simulink library "xrbsComm_r3"  (Simulink 5.1)
libraries: xbsIndex_r3 x775, xrbsComm_r3 x1
(part 4 of 6)

== system xrbsComm_r3/White Gaussian  Noise Generator/Box-Muller3/fr1/lfsr_41_2/x5 ==
  " " : Inport
  reset : Inport  Port=2
  ASR : Subsystem  mask{init=[init(9) init(8) init(7) init(6) init(5) init(4) init(3) init(2) init(1)]}
      mask prompts: init "Initial Value"
      mask init:
      | init_size = size(init);
      | asr_length = init_size(2);
  Register : xbsIndex_r3/Register  init=init(10)  reg_only_valid=off  explicit_period=on  period=-1  rst=on  en=off  out_en=off  dbl_ovrd=off
      settings: xl_area=[0, 0, 0, 0, 0, 0, 0]
  z-10 : Outport
  wires:
  Register/1 -> ASR/1(din)
  ASR/1(dout) -> z-10/1
  " "/1 -> Register/1
  reset/1 -> Register/2

== system xrbsComm_r3/White Gaussian  Noise Generator/Box-Muller3/fr1/lfsr_41_2/x6 ==
  " " : Inport
  reset : Inport  Port=2
  ASR : Subsystem  mask{init=[init(8) init(7) init(6) init(5) init(4) init(3) init(2) init(1)]}
      mask prompts: init "Initial Value"
      mask init:
      | init_size = size(init);
      | asr_length = init_size(2);
  Register1 : xbsIndex_r3/Register  init=init(9)  reg_only_valid=off  explicit_period=on  period=-1  rst=on  en=off  out_en=off  dbl_ovrd=off
      settings: xl_area=[0, 0, 0, 0, 0, 0, 0]
  z-9 : Outport
  wires:
  ASR/1(dout) -> z-9/1
  " "/1 -> Register1/1
  Register1/1 -> ASR/1(din)
  reset/1 -> Register1/2

== system xrbsComm_r3/White Gaussian  Noise Generator/Box-Muller3/fr1/lfsr_41_2/x7 ==
  " " : Inport
  reset : Inport  Port=2
  ASR : Subsystem  mask{init=[init(8) init(7) init(6) init(5) init(4) init(3) init(2) init(1)]}
      mask prompts: init "Initial Value"
      mask init:
      | init_size = size(init);
      | asr_length = init_size(2);
  Register1 : xbsIndex_r3/Register  init=init(9)  reg_only_valid=off  explicit_period=on  period=-1  rst=on  en=off  out_en=off  dbl_ovrd=off
      settings: xl_area=[0, 0, 0, 0, 0, 0, 0]
  z-9 : Outport
  wires:
  ASR/1(dout) -> z-9/1
  Register1/1 -> ASR/1(din)
  " "/1 -> Register1/1
  reset/1 -> Register1/2

== system xrbsComm_r3/White Gaussian  Noise Generator/Box-Muller3/g2/lfsr_47_5/x10 ==
  "  " : Inport
  reset : Inport  Port=2
  ASR : Subsystem  mask{init=[init(4) init(3) init(2) init(1)]}
      mask prompts: init "Initial Value"
      mask init:
      | init_size = size(init);
      | asr_length = init_size(2);
  Register5 : xbsIndex_r3/Register  init=init(5)  reg_only_valid=off  explicit_period=on  period=-1  rst=on  en=off  out_en=off  dbl_ovrd=off
      settings: xl_area=[0, 0, 0, 0, 0, 0, 0]
  z-5 : Outport
  wires:
  ASR/1(dout) -> z-5/1
  Register5/1 -> ASR/1(din)
  "  "/1 -> Register5/1
  reset/1 -> Register5/2

== system xrbsComm_r3/White Gaussian  Noise Generator/Box-Muller3/g2/lfsr_47_5/x11 ==
  " " : Inport
  reset : Inport  Port=2
  ASR : Subsystem  mask{init=[init(4) init(3) init(2) init(1)]}
      mask prompts: init "Initial Value"
      mask init:
      | init_size = size(init);
      | asr_length = init_size(2);
  Register : xbsIndex_r3/Register  init=init(5)  reg_only_valid=off  explicit_period=on  period=-1  rst=on  en=off  out_en=off  dbl_ovrd=off
      settings: xl_area=[0, 0, 0, 0, 0, 0, 0]
  z-5 : Outport
  wires:
  ASR/1(dout) -> z-5/1
  Register/1 -> ASR/1(din)
  " "/1 -> Register/1
  reset/1 -> Register/2

== system xrbsComm_r3/White Gaussian  Noise Generator/Box-Muller3/g2/lfsr_47_5/x12 ==
  " " : Inport
  reset : Inport  Port=2
  ASR : Subsystem  mask{init=[init(4) init(3) init(2) init(1)]}
      mask prompts: init "Initial Value"
      mask init:
      | init_size = size(init);
      | asr_length = init_size(2);
  Register : xbsIndex_r3/Register  init=init(5)  reg_only_valid=off  explicit_period=on  period=-1  rst=on  en=off  out_en=off  dbl_ovrd=off
      settings: xl_area=[0, 0, 0, 0, 0, 0, 0]
  z-5 : Outport
  wires:
  ASR/1(dout) -> z-5/1
  Register/1 -> ASR/1(din)
  " "/1 -> Register/1
  reset/1 -> Register/2

== system xrbsComm_r3/White Gaussian  Noise Generator/Box-Muller3/g2/lfsr_47_5/x13 ==
  note: reset
  " " : Inport
  " 1" : Inport  Port=2
  ASR : Subsystem  mask{init=[init(4) init(3) init(2) init(1)]}
      mask prompts: init "Initial Value"
      mask init:
      | init_size = size(init);
      | asr_length = init_size(2);
  Register : xbsIndex_r3/Register  init=init(5)  reg_only_valid=off  explicit_period=on  period=-1  rst=on  en=off  out_en=off  dbl_ovrd=off
      settings: xl_area=[0, 0, 0, 0, 0, 0, 0]
  z-5 : Outport
  wires:
  ASR/1(dout) -> z-5/1
  Register/1 -> ASR/1(din)
  " "/1 -> Register/1
  " 1"/1 -> Register/2

== system xrbsComm_r3/White Gaussian  Noise Generator/Box-Muller3/g2/lfsr_47_5/x14 ==
  " " : Inport
  reset : Inport  Port=2
  ASR : Subsystem  mask{init=[init(4) init(3) init(2) init(1)]}
      mask prompts: init "Initial Value"
      mask init:
      | init_size = size(init);
      | asr_length = init_size(2);
  Register : xbsIndex_r3/Register  init=init(5)  reg_only_valid=off  explicit_period=on  period=-1  rst=on  en=off  out_en=off  dbl_ovrd=off
      settings: xl_area=[0, 0, 0, 0, 0, 0, 0]
  z-5 : Outport
  wires:
  ASR/1(dout) -> z-5/1
  Register/1 -> ASR/1(din)
  " "/1 -> Register/1
  reset/1 -> Register/2

== system xrbsComm_r3/White Gaussian  Noise Generator/Box-Muller3/g2/lfsr_47_5/x15 ==
  " " : Inport
  reset : Inport  Port=2
  ASR : Subsystem  mask{init=[init(4) init(3) init(2) init(1)]}
      mask prompts: init "Initial Value"
      mask init:
      | init_size = size(init);
      | asr_length = init_size(2);
  Register : xbsIndex_r3/Register  init=init(5)  reg_only_valid=off  explicit_period=on  period=-1  rst=on  en=off  out_en=off  dbl_ovrd=off
      settings: xl_area=[0, 0, 0, 0, 0, 0, 0]
  z-5 : Outport
  wires:
  ASR/1(dout) -> z-5/1
  Register/1 -> ASR/1(din)
  " "/1 -> Register/1
  reset/1 -> Register/2

== system xrbsComm_r3/White Gaussian  Noise Generator/Box-Muller3/g2/lfsr_47_5/x16 ==
  " " : Inport
  reset : Inport  Port=2
  ASR : Subsystem  mask{init=[init(3) init(2) init(1)]}
      mask prompts: init "Initial Value"
      mask init:
      | init_size = size(init);
      | asr_length = init_size(2);
  Register : xbsIndex_r3/Register  init=init(4)  reg_only_valid=off  explicit_period=on  period=-1  rst=on  en=off  out_en=off  dbl_ovrd=off
      settings: xl_area=[0, 0, 0, 0, 0, 0, 0]
  z-4 : Outport
  wires:
  ASR/1(dout) -> z-4/1
  Register/1 -> ASR/1(din)
  " "/1 -> Register/1
  reset/1 -> Register/2

== system xrbsComm_r3/White Gaussian  Noise Generator/Box-Muller3/g2/lfsr_47_5/x9 ==
  " " : Inport
  reset : Inport  Port=2
  ASR : Subsystem  mask{init=[init(4) init(3) init(2) init(1)]}
      mask prompts: init "Initial Value"
      mask init:
      | init_size = size(init);
      | asr_length = init_size(2);
  Register : xbsIndex_r3/Register  init=init(5)  reg_only_valid=off  explicit_period=on  period=-1  rst=on  en=off  out_en=off  dbl_ovrd=off
      settings: xl_area=[0, 0, 0, 0, 0, 0, 0]
  z-5 : Outport
  wires:
  ASR/1(dout) -> z-5/1
  Register/1 -> ASR/1(din)
  " "/1 -> Register/1
  reset/1 -> Register/2

== system xrbsComm_r3/White Gaussian  Noise Generator/Box-Muller4/fr1/lfsr_17_2/x1 ==
  " " : Inport
  " reset" : Inport  Port=2
  ASR : Subsystem  mask{init=[init(2) init(1)]}
      mask prompts: init "Initial Value"
      mask init:
      | init_size = size(init);
      | asr_length = init_size(2);
  Register4 : xbsIndex_r3/Register  init=init(3)  reg_only_valid=off  explicit_period=on  period=-1  rst=on  en=off  out_en=off  dbl_ovrd=off
      settings: xl_area=[0, 0, 0, 0, 0, 0, 0]
  z-3 : Outport
  wires:
  " "/1 -> Register4/1
  ASR/1(dout) -> z-3/1
  Register4/1 -> ASR/1(din)
  " reset"/1 -> Register4/2

== system xrbsComm_r3/White Gaussian  Noise Generator/Box-Muller4/fr1/lfsr_17_2/x5 ==
  " " : Inport
  reset : Inport  Port=2
  ASR : Subsystem  mask{init=[init(3) init(2) init(1)]}
      mask prompts: init "Initial Value"
      mask init:
      | init_size = size(init);
      | asr_length = init_size(2);
  Register5 : xbsIndex_r3/Register  init=init(4)  reg_only_valid=off  explicit_period=on  period=-1  rst=on  en=off  out_en=off  dbl_ovrd=off
      settings: xl_area=[0, 0, 0, 0, 0, 0, 0]
  z-4 : Outport
  wires:
  ASR/1(dout) -> z-4/1
  Register5/1 -> ASR/1(din)
  " "/1 -> Register5/1
  reset/1 -> Register5/2

== system xrbsComm_r3/White Gaussian  Noise Generator/Box-Muller4/fr1/lfsr_17_2/x6 ==
  " " : Inport
  " reset" : Inport  Port=2
  ASR : Subsystem  mask{init=[init(2) init(1)]}
      mask prompts: init "Initial Value"
      mask init:
      | init_size = size(init);
      | asr_length = init_size(2);
  Register4 : xbsIndex_r3/Register  init=init(3)  reg_only_valid=off  explicit_period=on  period=-1  rst=on  en=off  out_en=off  dbl_ovrd=off
      settings: xl_area=[0, 0, 0, 0, 0, 0, 0]
  z-3 : Outport
  wires:
  ASR/1(dout) -> z-3/1
  " "/1 -> Register4/1
  Register4/1 -> ASR/1(din)
  " reset"/1 -> Register4/2

== system xrbsComm_r3/White Gaussian  Noise Generator/Box-Muller4/fr1/lfsr_17_2/x7 ==
  " " : Inport
  reset : Inport  Port=2
  ASR : Subsystem  mask{init=[init(2) init(1)]}
      mask prompts: init "Initial Value"
      mask init:
      | init_size = size(init);
      | asr_length = init_size(2);
  Register4 : xbsIndex_r3/Register  init=init(3)  reg_only_valid=off  explicit_period=on  period=-1  rst=on  en=off  out_en=off  dbl_ovrd=off
      settings: xl_area=[0, 0, 0, 0, 0, 0, 0]
  z-3 : Outport
  wires:
  " "/1 -> Register4/1
  ASR/1(dout) -> z-3/1
  Register4/1 -> ASR/1(din)
  reset/1 -> Register4/2

== system xrbsComm_r3/White Gaussian  Noise Generator/Box-Muller4/fr1/lfsr_25_2/x1 ==
  " " : Inport
  reset : Inport  Port=2
  ASR : Subsystem  mask{init=[init(4) init(3) init(2) init(1)]}
      mask prompts: init "Initial Value"
      mask init:
      | init_size = size(init);
      | asr_length = init_size(2);
  Register : xbsIndex_r3/Register  init=init(5)  reg_only_valid=off  explicit_period=on  period=-1  rst=on  en=off  out_en=off  dbl_ovrd=off
      settings: xl_area=[0, 0, 0, 0, 0, 0, 0]
  z-5 : Outport
  wires:
  Register/1 -> ASR/1(din)
  ASR/1(dout) -> z-5/1
  " "/1 -> Register/1
  reset/1 -> Register/2

== system xrbsComm_r3/White Gaussian  Noise Generator/Box-Muller4/fr1/lfsr_25_2/x5 ==
  " " : Inport
  reset : Inport  Port=2
  ASR : Subsystem  mask{init=[init(5) init(4) init(3) init(2) init(1)]}
      mask prompts: init "Initial Value"
      mask init:
      | init_size = size(init);
      | asr_length = init_size(2);
  Register : xbsIndex_r3/Register  init=init(6)  reg_only_valid=off  explicit_period=on  period=-1  rst=on  en=off  out_en=off  dbl_ovrd=off
      settings: xl_area=[0, 0, 0, 0, 0, 0, 0]
  z-6 : Outport
  wires:
  Register/1 -> ASR/1(din)
  ASR/1(dout) -> z-6/1
  " "/1 -> Register/1
  reset/1 -> Register/2

== system xrbsComm_r3/White Gaussian  Noise Generator/Box-Muller4/fr1/lfsr_25_2/x6 ==
  " " : Inport
  reset : Inport  Port=2
  ASR : Subsystem  mask{init=[init(4) init(3) init(2) init(1)]}
      mask prompts: init "Initial Value"
      mask init:
      | init_size = size(init);
      | asr_length = init_size(2);
  Register : xbsIndex_r3/Register  init=init(5)  reg_only_valid=off  explicit_period=on  period=-1  rst=on  en=off  out_en=off  dbl_ovrd=off
      settings: xl_area=[0, 0, 0, 0, 0, 0, 0]
  z-5 : Outport
  wires:
  Register/1 -> ASR/1(din)
  ASR/1(dout) -> z-5/1
  " "/1 -> Register/1
  reset/1 -> Register/2

== system xrbsComm_r3/White Gaussian  Noise Generator/Box-Muller4/fr1/lfsr_25_2/x7 ==
  " " : Inport
  reset : Inport  Port=2
  ASR : Subsystem  mask{init=[init(4) init(3) init(2) init(1)]}
      mask prompts: init "Initial Value"
      mask init:
      | init_size = size(init);
      | asr_length = init_size(2);
  Register : xbsIndex_r3/Register  init=init(5)  reg_only_valid=off  explicit_period=on  period=-1  rst=on  en=off  out_en=off  dbl_ovrd=off
      settings: xl_area=[0, 0, 0, 0, 0, 0, 0]
  z-5 : Outport
  wires:
  Register/1 -> ASR/1(din)
  ASR/1(dout) -> z-5/1
  " "/1 -> Register/1
  reset/1 -> Register/2

== system xrbsComm_r3/White Gaussian  Noise Generator/Box-Muller4/fr1/lfsr_29_2/x5 ==
  " " : Inport
  reset : Inport  Port=2
  ASR : Subsystem  mask{init=[init(6) init(5) init(4) init(3) init(2) init(1)]}
      mask prompts: init "Initial Value"
      mask init:
      | init_size = size(init);
      | asr_length = init_size(2);
  Register : xbsIndex_r3/Register  init=init(7)  reg_only_valid=off  explicit_period=on  period=-1  rst=on  en=off  out_en=off  dbl_ovrd=off
      settings: xl_area=[0, 0, 0, 0, 0, 0, 0]
  z-7 : Outport
  wires:
  ASR/1(dout) -> z-7/1
  Register/1 -> ASR/1(din)
  " "/1 -> Register/1
  reset/1 -> Register/2

== system xrbsComm_r3/White Gaussian  Noise Generator/Box-Muller4/fr1/lfsr_29_2/x6 ==
  " " : Inport
  reset : Inport  Port=2
  ASR : Subsystem  mask{init=[init(5) init(4) init(3) init(2) init(1)]}
      mask prompts: init "Initial Value"
      mask init:
      | init_size = size(init);
      | asr_length = init_size(2);
  Register : xbsIndex_r3/Register  init=init(6)  reg_only_valid=off  explicit_period=on  period=-1  rst=on  en=off  out_en=off  dbl_ovrd=off
      settings: xl_area=[0, 0, 0, 0, 0, 0, 0]
  z-6 : Outport
  wires:
  ASR/1(dout) -> z-6/1
  Register/1 -> ASR/1(din)
  " "/1 -> Register/1
  reset/1 -> Register/2

== system xrbsComm_r3/White Gaussian  Noise Generator/Box-Muller4/fr1/lfsr_29_2/x7 ==
  " " : Inport
  reset : Inport  Port=2
  ASR : Subsystem  mask{init=[init(5) init(4) init(3) init(2) init(1)]}
      mask prompts: init "Initial Value"
      mask init:
      | init_size = size(init);
      | asr_length = init_size(2);
  Register : xbsIndex_r3/Register  init=init(6)  reg_only_valid=off  explicit_period=on  period=-1  rst=on  en=off  out_en=off  dbl_ovrd=off
      settings: xl_area=[0, 0, 0, 0, 0, 0, 0]
  z-6 : Outport
  wires:
  ASR/1(dout) -> z-6/1
  Register/1 -> ASR/1(din)
  " "/1 -> Register/1
  reset/1 -> Register/2

== system xrbsComm_r3/White Gaussian  Noise Generator/Box-Muller4/fr1/lfsr_29_2/x8 ==
  " " : Inport
  reset : Inport  Port=2
  ASR : Subsystem  mask{init=[init(5) init(4) init(3) init(2) init(1)]}
      mask prompts: init "Initial Value"
      mask init:
      | init_size = size(init);
      | asr_length = init_size(2);
  Register : xbsIndex_r3/Register  init=init(6)  reg_only_valid=off  explicit_period=on  period=-1  rst=on  en=off  out_en=off  dbl_ovrd=off
      settings: xl_area=[0, 0, 0, 0, 0, 0, 0]
  z-6 : Outport
  wires:
  ASR/1(dout) -> z-6/1
  Register/1 -> ASR/1(din)
  " "/1 -> Register/1
  reset/1 -> Register/2

== system xrbsComm_r3/White Gaussian  Noise Generator/Box-Muller4/fr1/lfsr_31_2/x5 ==
  " " : Inport
  reset : Inport  Port=2
  ASR : Subsystem  mask{init=[init(6) init(5) init(4) init(3) init(2) init(1)]}
      mask prompts: init "Initial Value"
      mask init:
      | init_size = size(init);
      | asr_length = init_size(2);
  Register : xbsIndex_r3/Register  init=init(7)  reg_only_valid=off  explicit_period=on  period=-1  rst=on  en=off  out_en=off  dbl_ovrd=off
      settings: xl_area=[0, 0, 0, 0, 0, 0, 0]
  z-7 : Outport
  wires:
  Register/1 -> ASR/1(din)
  ASR/1(dout) -> z-7/1
  " "/1 -> Register/1
  reset/1 -> Register/2

== system xrbsComm_r3/White Gaussian  Noise Generator/Box-Muller4/fr1/lfsr_31_2/x6 ==
  " " : Inport
  reset : Inport  Port=2
  ASR : Subsystem  mask{init=[init(6) init(5) init(4) init(3) init(2) init(1)]}
      mask prompts: init "Initial Value"
      mask init:
      | init_size = size(init);
      | asr_length = init_size(2);
  Register : xbsIndex_r3/Register  init=init(7)  reg_only_valid=off  explicit_period=on  period=-1  rst=on  en=off  out_en=off  dbl_ovrd=off
      settings: xl_area=[0, 0, 0, 0, 0, 0, 0]
  z-7 : Outport
  wires:
  Register/1 -> ASR/1(din)
  " "/1 -> Register/1
  ASR/1(dout) -> z-7/1
  reset/1 -> Register/2

== system xrbsComm_r3/White Gaussian  Noise Generator/Box-Muller4/fr1/lfsr_31_2/x7 ==
  " " : Inport
  reset : Inport  Port=2
  ASR : Subsystem  mask{init=[init(6) init(5) init(4) init(3) init(2) init(1)]}
      mask prompts: init "Initial Value"
      mask init:
      | init_size = size(init);
      | asr_length = init_size(2);
  Register : xbsIndex_r3/Register  init=init(7)  reg_only_valid=off  explicit_period=on  period=-1  rst=on  en=off  out_en=off  dbl_ovrd=off
      settings: xl_area=[0, 0, 0, 0, 0, 0, 0]
  z-7 : Outport
  wires:
  Register/1 -> ASR/1(din)
  ASR/1(dout) -> z-7/1
  " "/1 -> Register/1
  reset/1 -> Register/2

== system xrbsComm_r3/White Gaussian  Noise Generator/Box-Muller4/fr1/lfsr_31_2/x8 ==
  " " : Inport
  reset : Inport  Port=2
  ASR : Subsystem  mask{init=[init(5) init(4) init(3) init(2) init(1)]}
      mask prompts: init "Initial Value"
      mask init:
      | init_size = size(init);
      | asr_length = init_size(2);
  Register : xbsIndex_r3/Register  init=init(6)  reg_only_valid=off  explicit_period=on  period=-1  rst=on  en=off  out_en=off  dbl_ovrd=off
      settings: xl_area=[0, 0, 0, 0, 0, 0, 0]
  z-6 : Outport
  wires:
  Register/1 -> ASR/1(din)
  " "/1 -> Register/1
  ASR/1(dout) -> z-6/1
  reset/1 -> Register/2

== system xrbsComm_r3/White Gaussian  Noise Generator/Box-Muller4/fr1/lfsr_41_2/x1 ==
  " " : Inport
  reset : Inport  Port=2
  ASR : Subsystem  mask{init=[init(8) init(7) init(6) init(5) init(4) init(3) init(2) init(1)]}
      mask prompts: init "Initial Value"
      mask init:
      | init_size = size(init);
      | asr_length = init_size(2);
  Register1 : xbsIndex_r3/Register  init=init(9)  reg_only_valid=off  explicit_period=on  period=-1  rst=on  en=off  out_en=off  dbl_ovrd=off
      settings: xl_area=[0, 0, 0, 0, 0, 0, 0]
  z-9 : Outport
  wires:
  ASR/1(dout) -> z-9/1
  " "/1 -> Register1/1
  Register1/1 -> ASR/1(din)
  reset/1 -> Register1/2

== system xrbsComm_r3/White Gaussian  Noise Generator/Box-Muller4/fr1/lfsr_41_2/x5 ==
  " " : Inport
  reset : Inport  Port=2
  ASR : Subsystem  mask{init=[init(9) init(8) init(7) init(6) init(5) init(4) init(3) init(2) init(1)]}
      mask prompts: init "Initial Value"
      mask init:
      | init_size = size(init);
      | asr_length = init_size(2);
  Register : xbsIndex_r3/Register  init=init(10)  reg_only_valid=off  explicit_period=on  period=-1  rst=on  en=off  out_en=off  dbl_ovrd=off
      settings: xl_area=[0, 0, 0, 0, 0, 0, 0]
  z-10 : Outport
  wires:
  Register/1 -> ASR/1(din)
  ASR/1(dout) -> z-10/1
  " "/1 -> Register/1
  reset/1 -> Register/2

== system xrbsComm_r3/White Gaussian  Noise Generator/Box-Muller4/fr1/lfsr_41_2/x6 ==
  " " : Inport
  reset : Inport  Port=2
  ASR : Subsystem  mask{init=[init(8) init(7) init(6) init(5) init(4) init(3) init(2) init(1)]}
      mask prompts: init "Initial Value"
      mask init:
      | init_size = size(init);
      | asr_length = init_size(2);
  Register1 : xbsIndex_r3/Register  init=init(9)  reg_only_valid=off  explicit_period=on  period=-1  rst=on  en=off  out_en=off  dbl_ovrd=off
      settings: xl_area=[0, 0, 0, 0, 0, 0, 0]
  z-9 : Outport
  wires:
  ASR/1(dout) -> z-9/1
  " "/1 -> Register1/1
  Register1/1 -> ASR/1(din)
  reset/1 -> Register1/2

== system xrbsComm_r3/White Gaussian  Noise Generator/Box-Muller4/fr1/lfsr_41_2/x7 ==
  " " : Inport
  reset : Inport  Port=2
  ASR : Subsystem  mask{init=[init(8) init(7) init(6) init(5) init(4) init(3) init(2) init(1)]}
      mask prompts: init "Initial Value"
      mask init:
      | init_size = size(init);
      | asr_length = init_size(2);
  Register1 : xbsIndex_r3/Register  init=init(9)  reg_only_valid=off  explicit_period=on  period=-1  rst=on  en=off  out_en=off  dbl_ovrd=off
      settings: xl_area=[0, 0, 0, 0, 0, 0, 0]
  z-9 : Outport
  wires:
  ASR/1(dout) -> z-9/1
  Register1/1 -> ASR/1(din)
  " "/1 -> Register1/1
  reset/1 -> Register1/2

== system xrbsComm_r3/White Gaussian  Noise Generator/Box-Muller4/g2/lfsr_47_5/x10 ==
  "  " : Inport
  reset : Inport  Port=2
  ASR : Subsystem  mask{init=[init(4) init(3) init(2) init(1)]}
      mask prompts: init "Initial Value"
      mask init:
      | init_size = size(init);
      | asr_length = init_size(2);
  Register5 : xbsIndex_r3/Register  init=init(5)  reg_only_valid=off  explicit_period=on  period=-1  rst=on  en=off  out_en=off  dbl_ovrd=off
      settings: xl_area=[0, 0, 0, 0, 0, 0, 0]
  z-5 : Outport
  wires:
  ASR/1(dout) -> z-5/1
  Register5/1 -> ASR/1(din)
  "  "/1 -> Register5/1
  reset/1 -> Register5/2

== system xrbsComm_r3/White Gaussian  Noise Generator/Box-Muller4/g2/lfsr_47_5/x11 ==
  " " : Inport
  reset : Inport  Port=2
  ASR : Subsystem  mask{init=[init(4) init(3) init(2) init(1)]}
      mask prompts: init "Initial Value"
      mask init:
      | init_size = size(init);
      | asr_length = init_size(2);
  Register : xbsIndex_r3/Register  init=init(5)  reg_only_valid=off  explicit_period=on  period=-1  rst=on  en=off  out_en=off  dbl_ovrd=off
      settings: xl_area=[0, 0, 0, 0, 0, 0, 0]
  z-5 : Outport
  wires:
  ASR/1(dout) -> z-5/1
  Register/1 -> ASR/1(din)
  " "/1 -> Register/1
  reset/1 -> Register/2

== system xrbsComm_r3/White Gaussian  Noise Generator/Box-Muller4/g2/lfsr_47_5/x12 ==
  " " : Inport
  reset : Inport  Port=2
  ASR : Subsystem  mask{init=[init(4) init(3) init(2) init(1)]}
      mask prompts: init "Initial Value"
      mask init:
      | init_size = size(init);
      | asr_length = init_size(2);
  Register : xbsIndex_r3/Register  init=init(5)  reg_only_valid=off  explicit_period=on  period=-1  rst=on  en=off  out_en=off  dbl_ovrd=off
      settings: xl_area=[0, 0, 0, 0, 0, 0, 0]
  z-5 : Outport
  wires:
  ASR/1(dout) -> z-5/1
  Register/1 -> ASR/1(din)
  " "/1 -> Register/1
  reset/1 -> Register/2

== system xrbsComm_r3/White Gaussian  Noise Generator/Box-Muller4/g2/lfsr_47_5/x13 ==
  note: reset
  " " : Inport
  " 1" : Inport  Port=2
  ASR : Subsystem  mask{init=[init(4) init(3) init(2) init(1)]}
      mask prompts: init "Initial Value"
      mask init:
      | init_size = size(init);
      | asr_length = init_size(2);
  Register : xbsIndex_r3/Register  init=init(5)  reg_only_valid=off  explicit_period=on  period=-1  rst=on  en=off  out_en=off  dbl_ovrd=off
      settings: xl_area=[0, 0, 0, 0, 0, 0, 0]
  z-5 : Outport
  wires:
  ASR/1(dout) -> z-5/1
  Register/1 -> ASR/1(din)
  " "/1 -> Register/1
  " 1"/1 -> Register/2

== system xrbsComm_r3/White Gaussian  Noise Generator/Box-Muller4/g2/lfsr_47_5/x14 ==
  " " : Inport
  reset : Inport  Port=2
  ASR : Subsystem  mask{init=[init(4) init(3) init(2) init(1)]}
      mask prompts: init "Initial Value"
      mask init:
      | init_size = size(init);
      | asr_length = init_size(2);
  Register : xbsIndex_r3/Register  init=init(5)  reg_only_valid=off  explicit_period=on  period=-1  rst=on  en=off  out_en=off  dbl_ovrd=off
      settings: xl_area=[0, 0, 0, 0, 0, 0, 0]
  z-5 : Outport
  wires:
  ASR/1(dout) -> z-5/1
  Register/1 -> ASR/1(din)
  " "/1 -> Register/1
  reset/1 -> Register/2

== system xrbsComm_r3/White Gaussian  Noise Generator/Box-Muller4/g2/lfsr_47_5/x15 ==
  " " : Inport
  reset : Inport  Port=2
  ASR : Subsystem  mask{init=[init(4) init(3) init(2) init(1)]}
      mask prompts: init "Initial Value"
      mask init:
      | init_size = size(init);
      | asr_length = init_size(2);
  Register : xbsIndex_r3/Register  init=init(5)  reg_only_valid=off  explicit_period=on  period=-1  rst=on  en=off  out_en=off  dbl_ovrd=off
      settings: xl_area=[0, 0, 0, 0, 0, 0, 0]
  z-5 : Outport
  wires:
  ASR/1(dout) -> z-5/1
  Register/1 -> ASR/1(din)
  " "/1 -> Register/1
  reset/1 -> Register/2

== system xrbsComm_r3/White Gaussian  Noise Generator/Box-Muller4/g2/lfsr_47_5/x16 ==
  " " : Inport
  reset : Inport  Port=2
  ASR : Subsystem  mask{init=[init(3) init(2) init(1)]}
      mask prompts: init "Initial Value"
      mask init:
      | init_size = size(init);
      | asr_length = init_size(2);
  Register : xbsIndex_r3/Register  init=init(4)  reg_only_valid=off  explicit_period=on  period=-1  rst=on  en=off  out_en=off  dbl_ovrd=off
      settings: xl_area=[0, 0, 0, 0, 0, 0, 0]
  z-4 : Outport
  wires:
  ASR/1(dout) -> z-4/1
  Register/1 -> ASR/1(din)
  " "/1 -> Register/1
  reset/1 -> Register/2

== system xrbsComm_r3/White Gaussian  Noise Generator/Box-Muller4/g2/lfsr_47_5/x9 ==
  " " : Inport
  reset : Inport  Port=2
  ASR : Subsystem  mask{init=[init(4) init(3) init(2) init(1)]}
      mask prompts: init "Initial Value"
      mask init:
      | init_size = size(init);
      | asr_length = init_size(2);
  Register : xbsIndex_r3/Register  init=init(5)  reg_only_valid=off  explicit_period=on  period=-1  rst=on  en=off  out_en=off  dbl_ovrd=off
      settings: xl_area=[0, 0, 0, 0, 0, 0, 0]
  z-5 : Outport
  wires:
  ASR/1(dout) -> z-5/1
  Register/1 -> ASR/1(din)
  " "/1 -> Register/1
  reset/1 -> Register/2

== system xrbsComm_r3/White Gaussian  Noise Generator/Box-Muller1/f/lfsr_17_2/x1/ASR ==
  din : Inport
  Addressable Shift Register : xbsIndex_r3/Addressable Shift Register  infer_latency=off  depth=asr_length  initVector=init  explicit_period=off  period=-1  accept_only_valid=off  en=off  dbl_ovrd=off  gen_core=on  use_rpm=off
      settings: xl_area=[0, 0, 0, 0, 0, 0, 0]
  Constant1 : xbsIndex_r3/Constant  const=asr_length-1  arith_type=Unsigned  n_bits=size(dec2bin(asr_length-1),2)  bin_pt=0  explicit_period=off  period=1  dbl_ovrd=off
  dout : Outport
  wires:
  Constant1/1 -> Addressable Shift Register/2
  Addressable Shift Register/1 -> dout/1
  din/1 -> Addressable Shift Register/1

== system xrbsComm_r3/White Gaussian  Noise Generator/Box-Muller1/f/lfsr_17_2/x5/ASR ==
  din : Inport
  Addressable Shift Register : xbsIndex_r3/Addressable Shift Register  infer_latency=off  depth=asr_length  initVector=init  explicit_period=off  period=-1  accept_only_valid=off  en=off  dbl_ovrd=off  gen_core=on  use_rpm=off
      settings: xl_area=[0, 0, 0, 0, 0, 0, 0]
  Constant : xbsIndex_r3/Constant  const=asr_length-1  arith_type=Unsigned  n_bits=size(dec2bin(asr_length-1),2)  bin_pt=0  explicit_period=off  period=1  dbl_ovrd=off
  dout : Outport
  wires:
  Constant/1 -> Addressable Shift Register/2
  Addressable Shift Register/1 -> dout/1
  din/1 -> Addressable Shift Register/1

== system xrbsComm_r3/White Gaussian  Noise Generator/Box-Muller1/f/lfsr_17_2/x6/ASR ==
  din : Inport
  Addressable Shift Register : xbsIndex_r3/Addressable Shift Register  infer_latency=off  depth=asr_length  initVector=init  explicit_period=off  period=-1  accept_only_valid=off  en=off  dbl_ovrd=off  gen_core=on  use_rpm=off
      settings: xl_area=[0, 0, 0, 0, 0, 0, 0]
  Constant : xbsIndex_r3/Constant  const=asr_length-1  arith_type=Unsigned  n_bits=size(dec2bin(asr_length-1),2)  bin_pt=0  explicit_period=off  period=1  dbl_ovrd=off
  dout : Outport
  wires:
  Constant/1 -> Addressable Shift Register/2
  Addressable Shift Register/1 -> dout/1
  din/1 -> Addressable Shift Register/1

== system xrbsComm_r3/White Gaussian  Noise Generator/Box-Muller1/f/lfsr_17_2/x7/ASR ==
  din : Inport
  Addressable Shift Register : xbsIndex_r3/Addressable Shift Register  infer_latency=off  depth=asr_length  initVector=init  explicit_period=off  period=-1  accept_only_valid=off  en=off  dbl_ovrd=off  gen_core=on  use_rpm=off
      settings: xl_area=[0, 0, 0, 0, 0, 0, 0]
  Constant : xbsIndex_r3/Constant  const=asr_length-1  arith_type=Unsigned  n_bits=size(dec2bin(asr_length-1),2)  bin_pt=0  explicit_period=off  period=1  dbl_ovrd=off
  dout : Outport
  wires:
  Constant/1 -> Addressable Shift Register/2
  Addressable Shift Register/1 -> dout/1
  din/1 -> Addressable Shift Register/1

== system xrbsComm_r3/White Gaussian  Noise Generator/Box-Muller1/f/lfsr_25_1/x1/ASR ==
  din : Inport
  Addressable Shift Register : xbsIndex_r3/Addressable Shift Register  infer_latency=off  depth=asr_length  initVector=init  explicit_period=off  period=-1  accept_only_valid=off  en=off  dbl_ovrd=off  gen_core=on  use_rpm=off
      settings: xl_area=[0, 0, 0, 0, 0, 0, 0]
  Constant1 : xbsIndex_r3/Constant  const=asr_length-1  arith_type=Unsigned  n_bits=size(dec2bin(asr_length-1),2)  bin_pt=0  explicit_period=off  period=1  dbl_ovrd=off
  dout : Outport
  wires:
  Constant1/1 -> Addressable Shift Register/2
  Addressable Shift Register/1 -> dout/1
  din/1 -> Addressable Shift Register/1

== system xrbsComm_r3/White Gaussian  Noise Generator/Box-Muller1/f/lfsr_25_1/x5/ASR ==
  din : Inport
  Addressable Shift Register : xbsIndex_r3/Addressable Shift Register  infer_latency=off  depth=asr_length  initVector=init  explicit_period=off  period=-1  accept_only_valid=off  en=off  dbl_ovrd=off  gen_core=on  use_rpm=off
      settings: xl_area=[0, 0, 0, 0, 0, 0, 0]
  Constant1 : xbsIndex_r3/Constant  const=asr_length-1  arith_type=Unsigned  n_bits=size(dec2bin(asr_length-1),2)  bin_pt=0  explicit_period=off  period=1  dbl_ovrd=off
  dout : Outport
  wires:
  Constant1/1 -> Addressable Shift Register/2
  Addressable Shift Register/1 -> dout/1
  din/1 -> Addressable Shift Register/1

== system xrbsComm_r3/White Gaussian  Noise Generator/Box-Muller1/f/lfsr_25_1/x6/ASR ==
  din : Inport
  Addressable Shift Register : xbsIndex_r3/Addressable Shift Register  infer_latency=off  depth=asr_length  initVector=init  explicit_period=off  period=-1  accept_only_valid=off  en=off  dbl_ovrd=off  gen_core=on  use_rpm=off
      settings: xl_area=[0, 0, 0, 0, 0, 0, 0]
  Constant1 : xbsIndex_r3/Constant  const=asr_length-1  arith_type=Unsigned  n_bits=size(dec2bin(asr_length-1),2)  bin_pt=0  explicit_period=off  period=1  dbl_ovrd=off
  dout : Outport
  wires:
  Constant1/1 -> Addressable Shift Register/2
  Addressable Shift Register/1 -> dout/1
  din/1 -> Addressable Shift Register/1

== system xrbsComm_r3/White Gaussian  Noise Generator/Box-Muller1/f/lfsr_25_1/x7/ASR ==
  din : Inport
  Addressable Shift Register : xbsIndex_r3/Addressable Shift Register  infer_latency=off  depth=asr_length  initVector=init  explicit_period=off  period=-1  accept_only_valid=off  en=off  dbl_ovrd=off  gen_core=on  use_rpm=off
      settings: xl_area=[0, 0, 0, 0, 0, 0, 0]
  Constant1 : xbsIndex_r3/Constant  const=asr_length-1  arith_type=Unsigned  n_bits=size(dec2bin(asr_length-1),2)  bin_pt=0  explicit_period=off  period=1  dbl_ovrd=off
  dout : Outport
  wires:
  Constant1/1 -> Addressable Shift Register/2
  Addressable Shift Register/1 -> dout/1
  din/1 -> Addressable Shift Register/1

== system xrbsComm_r3/White Gaussian  Noise Generator/Box-Muller1/f/lfsr_29_2/x5/ASR ==
  din : Inport
  Addressable Shift Register : xbsIndex_r3/Addressable Shift Register  infer_latency=off  depth=asr_length  initVector=init  explicit_period=off  period=-1  accept_only_valid=off  en=off  dbl_ovrd=off  gen_core=on  use_rpm=off
      settings: xl_area=[0, 0, 0, 0, 0, 0, 0]
  Constant1 : xbsIndex_r3/Constant  const=asr_length-1  arith_type=Unsigned  n_bits=size(dec2bin(asr_length-1),2)  bin_pt=0  explicit_period=off  period=1  dbl_ovrd=off
  dout : Outport
  wires:
  Constant1/1 -> Addressable Shift Register/2
  Addressable Shift Register/1 -> dout/1
  din/1 -> Addressable Shift Register/1

== system xrbsComm_r3/White Gaussian  Noise Generator/Box-Muller1/f/lfsr_29_2/x6/ASR ==
  din : Inport
  Addressable Shift Register : xbsIndex_r3/Addressable Shift Register  infer_latency=off  depth=asr_length  initVector=init  explicit_period=off  period=-1  accept_only_valid=off  en=off  dbl_ovrd=off  gen_core=on  use_rpm=off
      settings: xl_area=[0, 0, 0, 0, 0, 0, 0]
  Constant1 : xbsIndex_r3/Constant  const=asr_length-1  arith_type=Unsigned  n_bits=size(dec2bin(asr_length-1),2)  bin_pt=0  explicit_period=off  period=1  dbl_ovrd=off
  dout : Outport
  wires:
  Constant1/1 -> Addressable Shift Register/2
  Addressable Shift Register/1 -> dout/1
  din/1 -> Addressable Shift Register/1

== system xrbsComm_r3/White Gaussian  Noise Generator/Box-Muller1/f/lfsr_29_2/x7/ASR ==
  din : Inport
  Addressable Shift Register : xbsIndex_r3/Addressable Shift Register  infer_latency=off  depth=asr_length  initVector=init  explicit_period=off  period=-1  accept_only_valid=off  en=off  dbl_ovrd=off  gen_core=on  use_rpm=off
      settings: xl_area=[0, 0, 0, 0, 0, 0, 0]
  Constant1 : xbsIndex_r3/Constant  const=asr_length-1  arith_type=Unsigned  n_bits=size(dec2bin(asr_length-1),2)  bin_pt=0  explicit_period=off  period=1  dbl_ovrd=off
  dout : Outport
  wires:
  Constant1/1 -> Addressable Shift Register/2
  Addressable Shift Register/1 -> dout/1
  din/1 -> Addressable Shift Register/1

== system xrbsComm_r3/White Gaussian  Noise Generator/Box-Muller1/f/lfsr_29_2/x8/ASR ==
  din : Inport
  Addressable Shift Register : xbsIndex_r3/Addressable Shift Register  infer_latency=off  depth=asr_length  initVector=init  explicit_period=off  period=-1  accept_only_valid=off  en=off  dbl_ovrd=off  gen_core=on  use_rpm=off
      settings: xl_area=[0, 0, 0, 0, 0, 0, 0]
  Constant1 : xbsIndex_r3/Constant  const=asr_length-1  arith_type=Unsigned  n_bits=size(dec2bin(asr_length-1),2)  bin_pt=0  explicit_period=off  period=1  dbl_ovrd=off
  dout : Outport
  wires:
  Constant1/1 -> Addressable Shift Register/2
  Addressable Shift Register/1 -> dout/1
  din/1 -> Addressable Shift Register/1

== system xrbsComm_r3/White Gaussian  Noise Generator/Box-Muller1/f/lfsr_31_2/x5/ASR ==
  din : Inport
  Addressable Shift Register : xbsIndex_r3/Addressable Shift Register  infer_latency=off  depth=asr_length  initVector=init  explicit_period=off  period=-1  accept_only_valid=off  en=off  dbl_ovrd=off  gen_core=on  use_rpm=off
      settings: xl_area=[0, 0, 0, 0, 0, 0, 0]
  Constant1 : xbsIndex_r3/Constant  const=asr_length-1  arith_type=Unsigned  n_bits=size(dec2bin(asr_length-1),2)  bin_pt=0  explicit_period=off  period=1  dbl_ovrd=off
  dout : Outport
  wires:
  Constant1/1 -> Addressable Shift Register/2
  Addressable Shift Register/1 -> dout/1
  din/1 -> Addressable Shift Register/1

== system xrbsComm_r3/White Gaussian  Noise Generator/Box-Muller1/f/lfsr_31_2/x6/ASR ==
  din : Inport
  Addressable Shift Register : xbsIndex_r3/Addressable Shift Register  infer_latency=off  depth=asr_length  initVector=init  explicit_period=off  period=-1  accept_only_valid=off  en=off  dbl_ovrd=off  gen_core=on  use_rpm=off
      settings: xl_area=[0, 0, 0, 0, 0, 0, 0]
  Constant1 : xbsIndex_r3/Constant  const=asr_length-1  arith_type=Unsigned  n_bits=size(dec2bin(asr_length-1),2)  bin_pt=0  explicit_period=off  period=1  dbl_ovrd=off
  dout : Outport
  wires:
  Constant1/1 -> Addressable Shift Register/2
  Addressable Shift Register/1 -> dout/1
  din/1 -> Addressable Shift Register/1

== system xrbsComm_r3/White Gaussian  Noise Generator/Box-Muller1/f/lfsr_31_2/x7/ASR ==
  din : Inport
  Addressable Shift Register : xbsIndex_r3/Addressable Shift Register  infer_latency=off  depth=asr_length  initVector=init  explicit_period=off  period=-1  accept_only_valid=off  en=off  dbl_ovrd=off  gen_core=on  use_rpm=off
      settings: xl_area=[0, 0, 0, 0, 0, 0, 0]
  Constant1 : xbsIndex_r3/Constant  const=asr_length-1  arith_type=Unsigned  n_bits=size(dec2bin(asr_length-1),2)  bin_pt=0  explicit_period=off  period=1  dbl_ovrd=off
  dout : Outport
  wires:
  Constant1/1 -> Addressable Shift Register/2
  Addressable Shift Register/1 -> dout/1
  din/1 -> Addressable Shift Register/1

== system xrbsComm_r3/White Gaussian  Noise Generator/Box-Muller1/f/lfsr_31_2/x8/ASR ==
  din : Inport
  Addressable Shift Register : xbsIndex_r3/Addressable Shift Register  infer_latency=off  depth=asr_length  initVector=init  explicit_period=off  period=-1  accept_only_valid=off  en=off  dbl_ovrd=off  gen_core=on  use_rpm=off
      settings: xl_area=[0, 0, 0, 0, 0, 0, 0]
  Constant1 : xbsIndex_r3/Constant  const=asr_length-1  arith_type=Unsigned  n_bits=size(dec2bin(asr_length-1),2)  bin_pt=0  explicit_period=off  period=1  dbl_ovrd=off
  dout : Outport
  wires:
  Constant1/1 -> Addressable Shift Register/2
  Addressable Shift Register/1 -> dout/1
  din/1 -> Addressable Shift Register/1

== system xrbsComm_r3/White Gaussian  Noise Generator/Box-Muller1/f/lfsr_41_2/x1/ASR ==
  din : Inport
  Addressable Shift Register : xbsIndex_r3/Addressable Shift Register  infer_latency=off  depth=asr_length  initVector=init  explicit_period=off  period=-1  accept_only_valid=off  en=off  dbl_ovrd=off  gen_core=on  use_rpm=off
      settings: xl_area=[0, 0, 0, 0, 0, 0, 0]
  Constant1 : xbsIndex_r3/Constant  const=asr_length-1  arith_type=Unsigned  n_bits=size(dec2bin(asr_length-1),2)  bin_pt=0  explicit_period=off  period=1  dbl_ovrd=off
  dout : Outport
  wires:
  Constant1/1 -> Addressable Shift Register/2
  Addressable Shift Register/1 -> dout/1
  din/1 -> Addressable Shift Register/1

== system xrbsComm_r3/White Gaussian  Noise Generator/Box-Muller1/f/lfsr_41_2/x5/ASR ==
  din : Inport
  Addressable Shift Register : xbsIndex_r3/Addressable Shift Register  infer_latency=off  depth=asr_length  initVector=init  explicit_period=off  period=-1  accept_only_valid=off  en=off  dbl_ovrd=off  gen_core=on  use_rpm=off
      settings: xl_area=[0, 0, 0, 0, 0, 0, 0]
  Constant1 : xbsIndex_r3/Constant  const=asr_length-1  arith_type=Unsigned  n_bits=size(dec2bin(asr_length-1),2)  bin_pt=0  explicit_period=off  period=1  dbl_ovrd=off
  dout : Outport
  wires:
  Constant1/1 -> Addressable Shift Register/2
  Addressable Shift Register/1 -> dout/1
  din/1 -> Addressable Shift Register/1

== system xrbsComm_r3/White Gaussian  Noise Generator/Box-Muller1/f/lfsr_41_2/x6/ASR ==
  din : Inport
  Addressable Shift Register : xbsIndex_r3/Addressable Shift Register  infer_latency=off  depth=asr_length  initVector=init  explicit_period=off  period=-1  accept_only_valid=off  en=off  dbl_ovrd=off  gen_core=on  use_rpm=off
      settings: xl_area=[0, 0, 0, 0, 0, 0, 0]
  Constant1 : xbsIndex_r3/Constant  const=asr_length-1  arith_type=Unsigned  n_bits=size(dec2bin(asr_length-1),2)  bin_pt=0  explicit_period=off  period=1  dbl_ovrd=off
  dout : Outport
  wires:
  Constant1/1 -> Addressable Shift Register/2
  Addressable Shift Register/1 -> dout/1
  din/1 -> Addressable Shift Register/1

== system xrbsComm_r3/White Gaussian  Noise Generator/Box-Muller1/f/lfsr_41_2/x7/ASR ==
  din : Inport
  Addressable Shift Register : xbsIndex_r3/Addressable Shift Register  infer_latency=off  depth=asr_length  initVector=init  explicit_period=off  period=-1  accept_only_valid=off  en=off  dbl_ovrd=off  gen_core=on  use_rpm=off
      settings: xl_area=[0, 0, 0, 0, 0, 0, 0]
  Constant1 : xbsIndex_r3/Constant  const=asr_length-1  arith_type=Unsigned  n_bits=size(dec2bin(asr_length-1),2)  bin_pt=0  explicit_period=off  period=1  dbl_ovrd=off
  dout : Outport
  wires:
  Constant1/1 -> Addressable Shift Register/2
  Addressable Shift Register/1 -> dout/1
  din/1 -> Addressable Shift Register/1

== system xrbsComm_r3/White Gaussian  Noise Generator/Box-Muller1/g/lfsr_47_5/x10/ASR ==
  din : Inport
  Addressable Shift Register : xbsIndex_r3/Addressable Shift Register  infer_latency=off  depth=asr_length  initVector=init  explicit_period=off  period=-1  accept_only_valid=off  en=off  dbl_ovrd=off  gen_core=on  use_rpm=off
      settings: xl_area=[0, 0, 0, 0, 0, 0, 0]
  Constant1 : xbsIndex_r3/Constant  const=asr_length-1  arith_type=Unsigned  n_bits=size(dec2bin(asr_length-1),2)  bin_pt=0  explicit_period=off  period=1  dbl_ovrd=off
  dout : Outport
  wires:
  Constant1/1 -> Addressable Shift Register/2
  Addressable Shift Register/1 -> dout/1
  din/1 -> Addressable Shift Register/1

== system xrbsComm_r3/White Gaussian  Noise Generator/Box-Muller1/g/lfsr_47_5/x11/ASR ==
  din : Inport
  Addressable Shift Register : xbsIndex_r3/Addressable Shift Register  infer_latency=off  depth=asr_length  initVector=init  explicit_period=off  period=-1  accept_only_valid=off  en=off  dbl_ovrd=off  gen_core=on  use_rpm=off
      settings: xl_area=[0, 0, 0, 0, 0, 0, 0]
  Constant1 : xbsIndex_r3/Constant  const=asr_length-1  arith_type=Unsigned  n_bits=size(dec2bin(asr_length-1),2)  bin_pt=0  explicit_period=off  period=1  dbl_ovrd=off
  dout : Outport
  wires:
  Constant1/1 -> Addressable Shift Register/2
  Addressable Shift Register/1 -> dout/1
  din/1 -> Addressable Shift Register/1

== system xrbsComm_r3/White Gaussian  Noise Generator/Box-Muller1/g/lfsr_47_5/x12/ASR ==
  din : Inport
  Addressable Shift Register : xbsIndex_r3/Addressable Shift Register  infer_latency=off  depth=asr_length  initVector=init  explicit_period=off  period=-1  accept_only_valid=off  en=off  dbl_ovrd=off  gen_core=on  use_rpm=off
      settings: xl_area=[0, 0, 0, 0, 0, 0, 0]
  Constant1 : xbsIndex_r3/Constant  const=asr_length-1  arith_type=Unsigned  n_bits=size(dec2bin(asr_length-1),2)  bin_pt=0  explicit_period=off  period=1  dbl_ovrd=off
  dout : Outport
  wires:
  Constant1/1 -> Addressable Shift Register/2
  Addressable Shift Register/1 -> dout/1
  din/1 -> Addressable Shift Register/1

== system xrbsComm_r3/White Gaussian  Noise Generator/Box-Muller1/g/lfsr_47_5/x13/ASR ==
  din : Inport
  Addressable Shift Register : xbsIndex_r3/Addressable Shift Register  infer_latency=off  depth=asr_length  initVector=init  explicit_period=off  period=-1  accept_only_valid=off  en=off  dbl_ovrd=off  gen_core=on  use_rpm=off
      settings: xl_area=[0, 0, 0, 0, 0, 0, 0]
  Constant1 : xbsIndex_r3/Constant  const=asr_length-1  arith_type=Unsigned  n_bits=size(dec2bin(asr_length-1),2)  bin_pt=0  explicit_period=off  period=1  dbl_ovrd=off
  dout : Outport
  wires:
  Constant1/1 -> Addressable Shift Register/2
  Addressable Shift Register/1 -> dout/1
  din/1 -> Addressable Shift Register/1

== system xrbsComm_r3/White Gaussian  Noise Generator/Box-Muller1/g/lfsr_47_5/x14/ASR ==
  din : Inport
  Addressable Shift Register : xbsIndex_r3/Addressable Shift Register  infer_latency=off  depth=asr_length  initVector=init  explicit_period=off  period=-1  accept_only_valid=off  en=off  dbl_ovrd=off  gen_core=on  use_rpm=off
      settings: xl_area=[0, 0, 0, 0, 0, 0, 0]
  Constant1 : xbsIndex_r3/Constant  const=asr_length-1  arith_type=Unsigned  n_bits=size(dec2bin(asr_length-1),2)  bin_pt=0  explicit_period=off  period=1  dbl_ovrd=off
  dout : Outport
  wires:
  Constant1/1 -> Addressable Shift Register/2
  Addressable Shift Register/1 -> dout/1
  din/1 -> Addressable Shift Register/1

== system xrbsComm_r3/White Gaussian  Noise Generator/Box-Muller1/g/lfsr_47_5/x15/ASR ==
  din : Inport
  Addressable Shift Register : xbsIndex_r3/Addressable Shift Register  infer_latency=off  depth=asr_length  initVector=init  explicit_period=off  period=-1  accept_only_valid=off  en=off  dbl_ovrd=off  gen_core=on  use_rpm=off
      settings: xl_area=[0, 0, 0, 0, 0, 0, 0]
  Constant1 : xbsIndex_r3/Constant  const=asr_length-1  arith_type=Unsigned  n_bits=size(dec2bin(asr_length-1),2)  bin_pt=0  explicit_period=off  period=1  dbl_ovrd=off
  dout : Outport
  wires:
  Constant1/1 -> Addressable Shift Register/2
  Addressable Shift Register/1 -> dout/1
  din/1 -> Addressable Shift Register/1

== system xrbsComm_r3/White Gaussian  Noise Generator/Box-Muller1/g/lfsr_47_5/x16/ASR ==
  din : Inport
  Addressable Shift Register : xbsIndex_r3/Addressable Shift Register  infer_latency=off  depth=asr_length  initVector=init  explicit_period=off  period=-1  accept_only_valid=off  en=off  dbl_ovrd=off  gen_core=on  use_rpm=off
      settings: xl_area=[0, 0, 0, 0, 0, 0, 0]
  Constant1 : xbsIndex_r3/Constant  const=asr_length-1  arith_type=Unsigned  n_bits=size(dec2bin(asr_length-1),2)  bin_pt=0  explicit_period=off  period=1  dbl_ovrd=off
  dout : Outport
  wires:
  Constant1/1 -> Addressable Shift Register/2
  Addressable Shift Register/1 -> dout/1
  din/1 -> Addressable Shift Register/1

== system xrbsComm_r3/White Gaussian  Noise Generator/Box-Muller1/g/lfsr_47_5/x9/ASR ==
  din : Inport
  Addressable Shift Register : xbsIndex_r3/Addressable Shift Register  infer_latency=off  depth=asr_length  initVector=init  explicit_period=off  period=-1  accept_only_valid=off  en=off  dbl_ovrd=off  gen_core=on  use_rpm=off
      settings: xl_area=[0, 0, 0, 0, 0, 0, 0]
  Constant1 : xbsIndex_r3/Constant  const=asr_length-1  arith_type=Unsigned  n_bits=size(dec2bin(asr_length-1),2)  bin_pt=0  explicit_period=off  period=1  dbl_ovrd=off
  dout : Outport
  wires:
  Constant1/1 -> Addressable Shift Register/2
  Addressable Shift Register/1 -> dout/1
  din/1 -> Addressable Shift Register/1

== system xrbsComm_r3/White Gaussian  Noise Generator/Box-Muller2/fr1/lfsr_17_2/x1/ASR ==
  din : Inport
  Addressable Shift Register : xbsIndex_r3/Addressable Shift Register  infer_latency=off  depth=asr_length  initVector=init  explicit_period=off  period=-1  accept_only_valid=off  en=off  dbl_ovrd=off  gen_core=on  use_rpm=off
      settings: xl_area=[0, 0, 0, 0, 0, 0, 0]
  Constant : xbsIndex_r3/Constant  const=asr_length-1  arith_type=Unsigned  n_bits=size(dec2bin(asr_length-1),2)  bin_pt=0  explicit_period=off  period=1  dbl_ovrd=off
  dout : Outport
  wires:
  Constant/1 -> Addressable Shift Register/2
  Addressable Shift Register/1 -> dout/1
  din/1 -> Addressable Shift Register/1

== system xrbsComm_r3/White Gaussian  Noise Generator/Box-Muller2/fr1/lfsr_17_2/x5/ASR ==
  din : Inport
  Addressable Shift Register : xbsIndex_r3/Addressable Shift Register  infer_latency=off  depth=asr_length  initVector=init  explicit_period=off  period=-1  accept_only_valid=off  en=off  dbl_ovrd=off  gen_core=on  use_rpm=off
      settings: xl_area=[0, 0, 0, 0, 0, 0, 0]
  Constant1 : xbsIndex_r3/Constant  const=asr_length-1  arith_type=Unsigned  n_bits=size(dec2bin(asr_length-1),2)  bin_pt=0  explicit_period=off  period=1  dbl_ovrd=off
  dout : Outport
  wires:
  Constant1/1 -> Addressable Shift Register/2
  Addressable Shift Register/1 -> dout/1
  din/1 -> Addressable Shift Register/1

== system xrbsComm_r3/White Gaussian  Noise Generator/Box-Muller2/fr1/lfsr_17_2/x6/ASR ==
  din : Inport
  Addressable Shift Register : xbsIndex_r3/Addressable Shift Register  infer_latency=off  depth=asr_length  initVector=init  explicit_period=off  period=-1  accept_only_valid=off  en=off  dbl_ovrd=off  gen_core=on  use_rpm=off
      settings: xl_area=[0, 0, 0, 0, 0, 0, 0]
  Constant1 : xbsIndex_r3/Constant  const=asr_length-1  arith_type=Unsigned  n_bits=size(dec2bin(asr_length-1),2)  bin_pt=0  explicit_period=off  period=1  dbl_ovrd=off
  dout : Outport
  wires:
  Constant1/1 -> Addressable Shift Register/2
  Addressable Shift Register/1 -> dout/1
  din/1 -> Addressable Shift Register/1

== system xrbsComm_r3/White Gaussian  Noise Generator/Box-Muller2/fr1/lfsr_17_2/x7/ASR ==
  din : Inport
  Addressable Shift Register : xbsIndex_r3/Addressable Shift Register  infer_latency=off  depth=asr_length  initVector=init  explicit_period=off  period=-1  accept_only_valid=off  en=off  dbl_ovrd=off  gen_core=on  use_rpm=off
      settings: xl_area=[0, 0, 0, 0, 0, 0, 0]
  Constant1 : xbsIndex_r3/Constant  const=asr_length-1  arith_type=Unsigned  n_bits=size(dec2bin(asr_length-1),2)  bin_pt=0  explicit_period=off  period=1  dbl_ovrd=off
  dout : Outport
  wires:
  Constant1/1 -> Addressable Shift Register/2
  Addressable Shift Register/1 -> dout/1
  din/1 -> Addressable Shift Register/1

== system xrbsComm_r3/White Gaussian  Noise Generator/Box-Muller2/fr1/lfsr_25_2/x1/ASR ==
  din : Inport
  Addressable Shift Register : xbsIndex_r3/Addressable Shift Register  infer_latency=off  depth=asr_length  initVector=init  explicit_period=off  period=-1  accept_only_valid=off  en=off  dbl_ovrd=off  gen_core=on  use_rpm=off
      settings: xl_area=[0, 0, 0, 0, 0, 0, 0]
  Constant1 : xbsIndex_r3/Constant  const=asr_length-1  arith_type=Unsigned  n_bits=size(dec2bin(asr_length-1),2)  bin_pt=0  explicit_period=off  period=1  dbl_ovrd=off
  dout : Outport
  wires:
  Constant1/1 -> Addressable Shift Register/2
  Addressable Shift Register/1 -> dout/1
  din/1 -> Addressable Shift Register/1

== system xrbsComm_r3/White Gaussian  Noise Generator/Box-Muller2/fr1/lfsr_25_2/x5/ASR ==
  din : Inport
  Addressable Shift Register : xbsIndex_r3/Addressable Shift Register  infer_latency=off  depth=asr_length  initVector=init  explicit_period=off  period=-1  accept_only_valid=off  en=off  dbl_ovrd=off  gen_core=on  use_rpm=off
      settings: xl_area=[0, 0, 0, 0, 0, 0, 0]
  Constant1 : xbsIndex_r3/Constant  const=asr_length-1  arith_type=Unsigned  n_bits=size(dec2bin(asr_length-1),2)  bin_pt=0  explicit_period=off  period=1  dbl_ovrd=off
  dout : Outport
  wires:
  Constant1/1 -> Addressable Shift Register/2
  Addressable Shift Register/1 -> dout/1
  din/1 -> Addressable Shift Register/1

== system xrbsComm_r3/White Gaussian  Noise Generator/Box-Muller2/fr1/lfsr_25_2/x6/ASR ==
  din : Inport
  Addressable Shift Register : xbsIndex_r3/Addressable Shift Register  infer_latency=off  depth=asr_length  initVector=init  explicit_period=off  period=-1  accept_only_valid=off  en=off  dbl_ovrd=off  gen_core=on  use_rpm=off
      settings: xl_area=[0, 0, 0, 0, 0, 0, 0]
  Constant1 : xbsIndex_r3/Constant  const=asr_length-1  arith_type=Unsigned  n_bits=size(dec2bin(asr_length-1),2)  bin_pt=0  explicit_period=off  period=1  dbl_ovrd=off
  dout : Outport
  wires:
  Constant1/1 -> Addressable Shift Register/2
  Addressable Shift Register/1 -> dout/1
  din/1 -> Addressable Shift Register/1
